simulink model "DV3A_String1_Diode"  (R2023b)
settings: Solver=VariableStepAuto  StartTime=0.0  StopTime=1  FixedStep=Ts_Power  MinStep=0.0025  RelTol=1e-4
PreLoadFcn:
  | Ts_Power=5e-4;
  | Slope_Vdc=1;
InitFcn:
  | Ts_Power=50e-6;
  | Tc=1e-5;%break algebraic loop time constant
StopFcn:
  | if exist('I','var') && exist('V','var')
  |    figure(1)
  |    clf
  |    n=find(I>=0);
  |    n=n(end);
  |    Vglobal=V(1:n);
  |    Iglobal=I(1:n);
  | 
  | 
  |    Pglobal=Vglobal.*Iglobal;
  |    n=find(Pglobal==max(Pglobal));
  |    Pmax=Pglobal(n);
  |    Vmp=Vglobal(n);
  |    Imp=Iglobal(n);
  | 
  | 
  |    subplot(211)
  |    plot(Vglobal, Iglobal,Vmp,Imp,'or')
  |    ylabel('Current (A)')
  |    title(sprintf('Global I-V & P-V characteristics\n %s' ,ModuleName))
  | 
  | 
  |    subplot(212)
  |    plot(Vglobal, Pglobal,Vmp,Pmax,'or')
  |    ylabel('Power (W)')
  |    xlabel('Voltage (V)')
  | end
model workspace (MAT data in the model file):
  slope_Vdc = 3.0848387096
undefined symbols (not defined in the file): Slope_Vdc_string1
libraries: spsPVArrayLib x142, spsVariableResistorLib x142, spsDiodeLib x29, spsCurrentMeasurementLib x1, spsVoltageMeasurementLib x1, spsControlledVoltageSourceLib x1, simulink x1, spspowerguiLib x1
(part 1 of 8)
settings Model: Creator=MathWorks  LastModifiedBy=IT
settings SolverCC: AlgebraicLoopSolver=LineSearch
settings DataIOCC: ExternalInput=[]  LimitDataPoints=on  LoadExternalInput=on  SaveFormat=Array  SaveOutput=off  SignalLogging=off  DSMLogging=off  SaveTime=off  ReturnWorkspaceOutputs=off
settings OptimizationCC: ExpressionDepthLimit=2147483647  LifeSpan=inf
settings DebuggingCC: UnderspecifiedInitializationDetection=Classic  MergeDetectMultiDrivingBlocksExec=none  SolverPrmCheckMsg=warning  FcnCallInpInsideContextMsg=warning  UnconnectedInputMsg=warning  UnconnectedOutputMsg=warning  UnconnectedLineMsg=warning  AllowSymbolicDim=off  StateNameClashWarn=warning  SFUnexpectedBacktrackingDiag=warning  SFNoUnconditionalDefaultTransitionDiag=warning  SFExecutionAtInitializationDiag=none  ArithmeticOperatorsInVariantConditions=warning
settings HardwareCC: ProdBitPerPointer=32  ProdBitPerSizeT=32  ProdBitPerPtrDiffT=32  ProdLargestAtomicFloat=None  ProdIntDivRoundTo=Undefined  ProdEndianess=Unspecified  ProdWordSize=32  ProdHWDeviceType=32-bit Generic
settings ModelReferenceCC: EnableRefExpFcnMdlSchedulingChecks=on  PropagateSignalLabelsOutOfModel=off
settings SFSimCC: SimUseLocalCustomCode=off  CustomCodeUndefinedFunction=UseInterfaceOnly
settings RTWCC: RTWUseLocalCustomCode=off  DLArmComputeVersion=19.05
settings CodeAppCC: StateflowObjectComments=on
settings GRTTargetCC: TargetLangStandard=C89/C90 (ANSI)  CombineOutputUpdateFcns=off  GRTInterface=on
settings ConfigComp: CovMetricSettings=dw  CovSaveCumulativeToWorkspaceVar=on  CovSaveSingleToWorkspaceVar=on  CovExternalEMLEnable=off  CovSFcnEnable=off
settings SimscapeCC: SimscapeNormalizeSystem=off

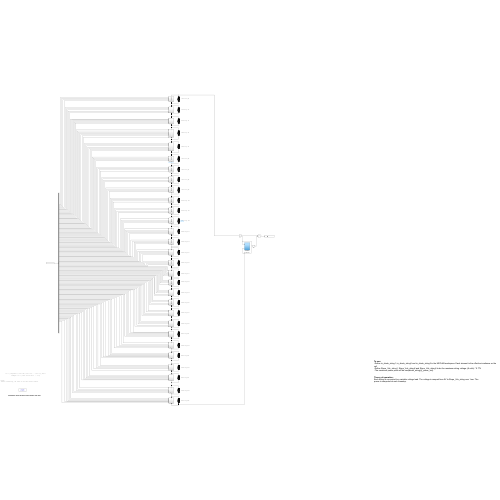
[thumbnail: Simulink's stored preview of the top-level diagram]
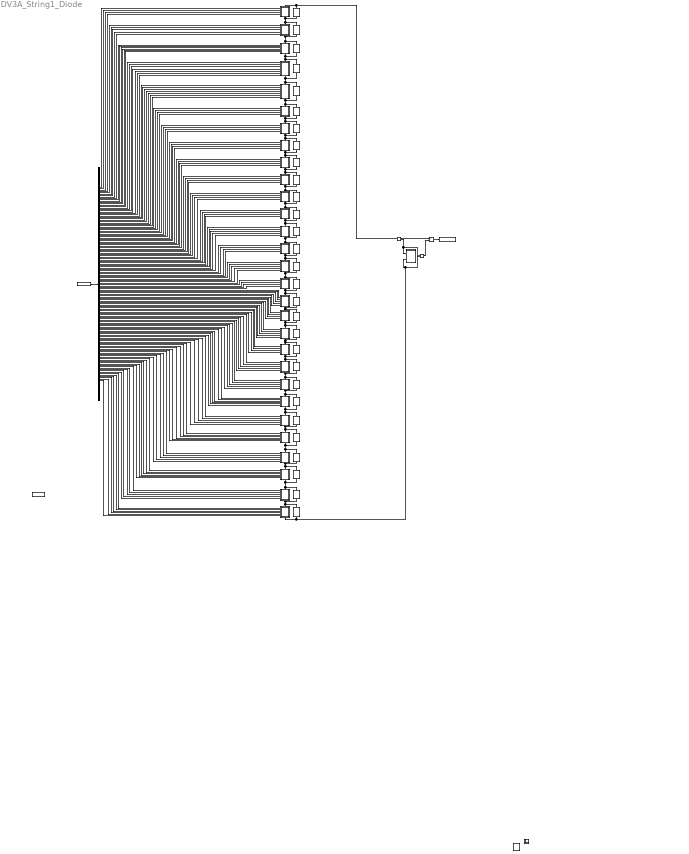
== system DV3A_String1_Diode ==
  note: irr = [(required 0) (cell 142) (cell 141) ... (cell 1)], W/m^2
  note: Notes:
      | -Within a substring, the order of the cells doesn't matter
  note: Final DV3A - String #1 with bypass diodes (142 cells)
  note: Example: irr = [0 800 700 242 573.3 ... 473]
  note: To use:
      | -Define irr_diode_string1, irr_diode_string2 and irr_diode_string3 in the MATLAB workspace. Each element is the effective irradiance on the cell
      | -Define Slope_Vdc_string1, Slope_Vdc_string2 and Slope_Vdc_string3 to be the maximum string voltage: (# cells) * 0.77V
      | -The maximum power point will be max(diode_string[n]_power_out )
  note: Theory of operation:
      | Each string is connected to a variable voltage load. The voltage is ramped from 0V to Slope_Vdc_string over 1sec. The power is computed at each timestep.
  note: Substring #1
  note: Substring #2
  note: Substring #3
  note: Substring #4
  note: Substring #5
  note: Substring #6
  note: Substring #7
  note: Substring #9
  note: Substring #8
  note: Substring #11
  note: Substring #10
  note: Substring #12
  note: Substring #13
  note: Substring #15
  note: Substring #14
  note: Substring #17
  note: Substring #16
  note: Substring #18
  note: Substring #19
  note: Substring #20
  note: Substring #21
  note: Substring #22
  note: Substring #23
  note: Substring #25
  note: Substring #24
  note: Substring #27
  note: Substring #26
  note: Substring #29
  note: Substring #28
  Bypass Diode {12..20,34..53} (29 alike) : spsDiodeLib/Diode  Ron=0.00333333  Lon=0  Vf=0.01993333134  IC=0  UseSnubber=off  Rs=1000000000  Cs=250e-15  Measurements=off
  Demux2 : Demux  Outputs=142
  From Workspace2 : FromWorkspace  VariableName=irr_diode_string_String1
  I1 : spsCurrentMeasurementLib/Current Measurement  PhasorSimulation=off  OutputType=Complex  PSBequivalent=0
  Product2 : Product
  Subsystem12 : Subsystem
      settings: PortSchema="{\"entries\":[{\"content\":{\"sides\":[{\"content\":{\"connectorIds\":[\"In1\",\"In2\",\"In3\",\"In4\"]},\"type\":\"ConnectorPlacement.EquallySpacedRectSide\",\"uuid\":\"ec6071b1-e44d-45a4-9204-34cda7b2c9be\"},{\"content\":{\"connectorIds\":[],\"side\":\"RIGHT\"},\"type\":\"ConnectorPlacement.EquallySpacedRectSide\",\"uuid\":\"8ac2ba72-278d-4942-985d-63a53d830fa7\"},{\"content\":{\"connectorIds\":[\"LConn1\"],\"side\":\"TOP\"},\"type\":\"ConnectorPlacement.EquallySpacedRectSide\",\"uuid\":\"91abef48-6106-4bba-9094-b5b4c6d4927b\"},{\"content\":{\"connectorIds\":[\"RConn1\"],\"side\":\"BOTTOM\"},\"type\":\"ConnectorPlacement.EquallySpacedRectSide\",\"uuid\":\"2339e630-2664-445f-8cd2-24ead5b760e5\"}]},\"type\":\"ConnectorPlacement.EquallySpacedConnector\",\"uuid\":\"6b30c10d-3aac-43c1-96cb-d205f04f2f88\"}],\"packageUris\":[\"http://schema.mathworks.com/mf0/Connector/R2020b\"],\"version\":\"1.0\"}"
  Subsystem13 : Subsystem
      settings: PortSchema="{\"entries\":[{\"content\":{\"sides\":[{\"content\":{\"connectorIds\":[\"In1\",\"In2\",\"In3\",\"In4\",\"In5\"]},\"type\":\"ConnectorPlacement.EquallySpacedRectSide\",\"uuid\":\"ec6071b1-e44d-45a4-9204-34cda7b2c9be\"},{\"content\":{\"side\":\"RIGHT\"},\"type\":\"ConnectorPlacement.EquallySpacedRectSide\",\"uuid\":\"8ac2ba72-278d-4942-985d-63a53d830fa7\"},{\"content\":{\"connectorIds\":[\"LConn1\"],\"side\":\"TOP\"},\"type\":\"ConnectorPlacement.EquallySpacedRectSide\",\"uuid\":\"91abef48-6106-4bba-9094-b5b4c6d4927b\"},{\"content\":{\"connectorIds\":[\"RConn1\"],\"side\":\"BOTTOM\"},\"type\":\"ConnectorPlacement.EquallySpacedRectSide\",\"uuid\":\"2339e630-2664-445f-8cd2-24ead5b760e5\"}]},\"type\":\"ConnectorPlacement.EquallySpacedConnector\",\"uuid\":\"6b30c10d-3aac-43c1-96cb-d205f04f2f88\"}],\"packageUris\":[\"http://schema.mathworks.com/mf0/Connector/R2020b\"],\"version\":\"1.0\"}"
  Subsystem14 : Subsystem
      settings: PortSchema="{\"entries\":[{\"content\":{\"sides\":[{\"content\":{\"connectorIds\":[\"In1\",\"In2\",\"In3\",\"In4\",\"In5\",\"In6\"]},\"type\":\"ConnectorPlacement.EquallySpacedRectSide\",\"uuid\":\"ec6071b1-e44d-45a4-9204-34cda7b2c9be\"},{\"content\":{\"side\":\"RIGHT\"},\"type\":\"ConnectorPlacement.EquallySpacedRectSide\",\"uuid\":\"8ac2ba72-278d-4942-985d-63a53d830fa7\"},{\"content\":{\"connectorIds\":[\"LConn1\"],\"side\":\"TOP\"},\"type\":\"ConnectorPlacement.EquallySpacedRectSide\",\"uuid\":\"91abef48-6106-4bba-9094-b5b4c6d4927b\"},{\"content\":{\"connectorIds\":[\"RConn1\"],\"side\":\"BOTTOM\"},\"type\":\"ConnectorPlacement.EquallySpacedRectSide\",\"uuid\":\"2339e630-2664-445f-8cd2-24ead5b760e5\"}]},\"type\":\"ConnectorPlacement.EquallySpacedConnector\",\"uuid\":\"6b30c10d-3aac-43c1-96cb-d205f04f2f88\"}],\"packageUris\":[\"http://schema.mathworks.com/mf0/Connector/R2020b\"],\"version\":\"1.0\"}"
  Subsystem15 : Subsystem
      settings: PortSchema="{\"entries\":[{\"content\":{\"sides\":[{\"content\":{\"connectorIds\":[\"In1\",\"In2\",\"In3\",\"In4\",\"In5\",\"In6\",\"In7\"]},\"type\":\"ConnectorPlacement.EquallySpacedRectSide\",\"uuid\":\"ec6071b1-e44d-45a4-9204-34cda7b2c9be\"},{\"content\":{\"connectorIds\":[],\"side\":\"RIGHT\"},\"type\":\"ConnectorPlacement.EquallySpacedRectSide\",\"uuid\":\"8ac2ba72-278d-4942-985d-63a53d830fa7\"},{\"content\":{\"connectorIds\":[\"LConn1\"],\"side\":\"TOP\"},\"type\":\"ConnectorPlacement.EquallySpacedRectSide\",\"uuid\":\"91abef48-6106-4bba-9094-b5b4c6d4927b\"},{\"content\":{\"connectorIds\":[\"RConn1\"],\"side\":\"BOTTOM\"},\"type\":\"ConnectorPlacement.EquallySpacedRectSide\",\"uuid\":\"2339e630-2664-445f-8cd2-24ead5b760e5\"}]},\"type\":\"ConnectorPlacement.EquallySpacedConnector\",\"uuid\":\"6b30c10d-3aac-43c1-96cb-d205f04f2f88\"}],\"packageUris\":[\"http://schema.mathworks.com/mf0/Connector/R2020b\"],\"version\":\"1.0\"}"
  Subsystem16 : Subsystem
      settings: PortSchema="{\"entries\":[{\"content\":{\"sides\":[{\"content\":{\"connectorIds\":[\"In1\",\"In2\",\"In3\",\"In4\",\"In5\",\"In6\",\"In7\"]},\"type\":\"ConnectorPlacement.EquallySpacedRectSide\",\"uuid\":\"ec6071b1-e44d-45a4-9204-34cda7b2c9be\"},{\"content\":{\"connectorIds\":[],\"side\":\"RIGHT\"},\"type\":\"ConnectorPlacement.EquallySpacedRectSide\",\"uuid\":\"8ac2ba72-278d-4942-985d-63a53d830fa7\"},{\"content\":{\"connectorIds\":[\"LConn1\"],\"side\":\"TOP\"},\"type\":\"ConnectorPlacement.EquallySpacedRectSide\",\"uuid\":\"91abef48-6106-4bba-9094-b5b4c6d4927b\"},{\"content\":{\"connectorIds\":[\"RConn1\"],\"side\":\"BOTTOM\"},\"type\":\"ConnectorPlacement.EquallySpacedRectSide\",\"uuid\":\"2339e630-2664-445f-8cd2-24ead5b760e5\"}]},\"type\":\"ConnectorPlacement.EquallySpacedConnector\",\"uuid\":\"6b30c10d-3aac-43c1-96cb-d205f04f2f88\"}],\"packageUris\":[\"http://schema.mathworks.com/mf0/Connector/R2020b\"],\"version\":\"1.0\"}"
  Subsystem17 : Subsystem
      settings: PortSchema="{\"entries\":[{\"content\":{\"sides\":[{\"content\":{\"connectorIds\":[\"In1\",\"In2\",\"In3\",\"In4\"]},\"type\":\"ConnectorPlacement.EquallySpacedRectSide\",\"uuid\":\"ec6071b1-e44d-45a4-9204-34cda7b2c9be\"},{\"content\":{\"connectorIds\":[],\"side\":\"RIGHT\"},\"type\":\"ConnectorPlacement.EquallySpacedRectSide\",\"uuid\":\"8ac2ba72-278d-4942-985d-63a53d830fa7\"},{\"content\":{\"connectorIds\":[\"LConn1\"],\"side\":\"TOP\"},\"type\":\"ConnectorPlacement.EquallySpacedRectSide\",\"uuid\":\"91abef48-6106-4bba-9094-b5b4c6d4927b\"},{\"content\":{\"connectorIds\":[\"RConn1\"],\"side\":\"BOTTOM\"},\"type\":\"ConnectorPlacement.EquallySpacedRectSide\",\"uuid\":\"2339e630-2664-445f-8cd2-24ead5b760e5\"}]},\"type\":\"ConnectorPlacement.EquallySpacedConnector\",\"uuid\":\"6b30c10d-3aac-43c1-96cb-d205f04f2f88\"}],\"packageUris\":[\"http://schema.mathworks.com/mf0/Connector/R2020b\"],\"version\":\"1.0\"}"
  Subsystem18 : Subsystem
      settings: PortSchema="{\"entries\":[{\"content\":{\"sides\":[{\"content\":{\"connectorIds\":[\"In1\",\"In2\",\"In3\",\"In4\"]},\"type\":\"ConnectorPlacement.EquallySpacedRectSide\",\"uuid\":\"ec6071b1-e44d-45a4-9204-34cda7b2c9be\"},{\"content\":{\"connectorIds\":[],\"side\":\"RIGHT\"},\"type\":\"ConnectorPlacement.EquallySpacedRectSide\",\"uuid\":\"8ac2ba72-278d-4942-985d-63a53d830fa7\"},{\"content\":{\"connectorIds\":[\"LConn1\"],\"side\":\"TOP\"},\"type\":\"ConnectorPlacement.EquallySpacedRectSide\",\"uuid\":\"91abef48-6106-4bba-9094-b5b4c6d4927b\"},{\"content\":{\"connectorIds\":[\"RConn1\"],\"side\":\"BOTTOM\"},\"type\":\"ConnectorPlacement.EquallySpacedRectSide\",\"uuid\":\"2339e630-2664-445f-8cd2-24ead5b760e5\"}]},\"type\":\"ConnectorPlacement.EquallySpacedConnector\",\"uuid\":\"6b30c10d-3aac-43c1-96cb-d205f04f2f88\"}],\"packageUris\":[\"http://schema.mathworks.com/mf0/Connector/R2020b\"],\"version\":\"1.0\"}"
  Subsystem19 : Subsystem
      settings: PortSchema="{\"entries\":[{\"content\":{\"sides\":[{\"content\":{\"connectorIds\":[\"In1\",\"In2\",\"In3\",\"In4\"]},\"type\":\"ConnectorPlacement.EquallySpacedRectSide\",\"uuid\":\"ec6071b1-e44d-45a4-9204-34cda7b2c9be\"},{\"content\":{\"connectorIds\":[],\"side\":\"RIGHT\"},\"type\":\"ConnectorPlacement.EquallySpacedRectSide\",\"uuid\":\"8ac2ba72-278d-4942-985d-63a53d830fa7\"},{\"content\":{\"connectorIds\":[\"LConn1\"],\"side\":\"TOP\"},\"type\":\"ConnectorPlacement.EquallySpacedRectSide\",\"uuid\":\"91abef48-6106-4bba-9094-b5b4c6d4927b\"},{\"content\":{\"connectorIds\":[\"RConn1\"],\"side\":\"BOTTOM\"},\"type\":\"ConnectorPlacement.EquallySpacedRectSide\",\"uuid\":\"2339e630-2664-445f-8cd2-24ead5b760e5\"}]},\"type\":\"ConnectorPlacement.EquallySpacedConnector\",\"uuid\":\"6b30c10d-3aac-43c1-96cb-d205f04f2f88\"}],\"packageUris\":[\"http://schema.mathworks.com/mf0/Connector/R2020b\"],\"version\":\"1.0\"}"
  Subsystem20 : Subsystem
      settings: PortSchema="{\"entries\":[{\"content\":{\"sides\":[{\"content\":{\"connectorIds\":[\"In1\",\"In2\",\"In3\",\"In4\"]},\"type\":\"ConnectorPlacement.EquallySpacedRectSide\",\"uuid\":\"ec6071b1-e44d-45a4-9204-34cda7b2c9be\"},{\"content\":{\"connectorIds\":[],\"side\":\"RIGHT\"},\"type\":\"ConnectorPlacement.EquallySpacedRectSide\",\"uuid\":\"8ac2ba72-278d-4942-985d-63a53d830fa7\"},{\"content\":{\"connectorIds\":[\"LConn1\"],\"side\":\"TOP\"},\"type\":\"ConnectorPlacement.EquallySpacedRectSide\",\"uuid\":\"91abef48-6106-4bba-9094-b5b4c6d4927b\"},{\"content\":{\"connectorIds\":[\"RConn1\"],\"side\":\"BOTTOM\"},\"type\":\"ConnectorPlacement.EquallySpacedRectSide\",\"uuid\":\"2339e630-2664-445f-8cd2-24ead5b760e5\"}]},\"type\":\"ConnectorPlacement.EquallySpacedConnector\",\"uuid\":\"6b30c10d-3aac-43c1-96cb-d205f04f2f88\"}],\"packageUris\":[\"http://schema.mathworks.com/mf0/Connector/R2020b\"],\"version\":\"1.0\"}"
  Subsystem34 : Subsystem
      settings: PortSchema="{\"entries\":[{\"content\":{\"sides\":[{\"content\":{\"connectorIds\":[\"In1\",\"In2\",\"In3\",\"In4\"]},\"type\":\"ConnectorPlacement.EquallySpacedRectSide\",\"uuid\":\"ec6071b1-e44d-45a4-9204-34cda7b2c9be\"},{\"content\":{\"connectorIds\":[],\"side\":\"RIGHT\"},\"type\":\"ConnectorPlacement.EquallySpacedRectSide\",\"uuid\":\"8ac2ba72-278d-4942-985d-63a53d830fa7\"},{\"content\":{\"connectorIds\":[\"LConn1\"],\"side\":\"TOP\"},\"type\":\"ConnectorPlacement.EquallySpacedRectSide\",\"uuid\":\"91abef48-6106-4bba-9094-b5b4c6d4927b\"},{\"content\":{\"connectorIds\":[\"RConn1\"],\"side\":\"BOTTOM\"},\"type\":\"ConnectorPlacement.EquallySpacedRectSide\",\"uuid\":\"2339e630-2664-445f-8cd2-24ead5b760e5\"}]},\"type\":\"ConnectorPlacement.EquallySpacedConnector\",\"uuid\":\"6b30c10d-3aac-43c1-96cb-d205f04f2f88\"}],\"packageUris\":[\"http://schema.mathworks.com/mf0/Connector/R2020b\"],\"version\":\"1.0\"}"
  Subsystem35 : Subsystem
      settings: PortSchema="{\"entries\":[{\"content\":{\"sides\":[{\"content\":{\"connectorIds\":[\"In1\",\"In2\",\"In3\",\"In4\"]},\"type\":\"ConnectorPlacement.EquallySpacedRectSide\",\"uuid\":\"ec6071b1-e44d-45a4-9204-34cda7b2c9be\"},{\"content\":{\"connectorIds\":[],\"side\":\"RIGHT\"},\"type\":\"ConnectorPlacement.EquallySpacedRectSide\",\"uuid\":\"8ac2ba72-278d-4942-985d-63a53d830fa7\"},{\"content\":{\"connectorIds\":[\"LConn1\"],\"side\":\"TOP\"},\"type\":\"ConnectorPlacement.EquallySpacedRectSide\",\"uuid\":\"91abef48-6106-4bba-9094-b5b4c6d4927b\"},{\"content\":{\"connectorIds\":[\"RConn1\"],\"side\":\"BOTTOM\"},\"type\":\"ConnectorPlacement.EquallySpacedRectSide\",\"uuid\":\"2339e630-2664-445f-8cd2-24ead5b760e5\"}]},\"type\":\"ConnectorPlacement.EquallySpacedConnector\",\"uuid\":\"6b30c10d-3aac-43c1-96cb-d205f04f2f88\"}],\"packageUris\":[\"http://schema.mathworks.com/mf0/Connector/R2020b\"],\"version\":\"1.0\"}"
  Subsystem36 : Subsystem
      settings: PortSchema="{\"entries\":[{\"content\":{\"sides\":[{\"content\":{\"connectorIds\":[\"In1\",\"In2\",\"In3\",\"In4\"]},\"type\":\"ConnectorPlacement.EquallySpacedRectSide\",\"uuid\":\"ec6071b1-e44d-45a4-9204-34cda7b2c9be\"},{\"content\":{\"connectorIds\":[],\"side\":\"RIGHT\"},\"type\":\"ConnectorPlacement.EquallySpacedRectSide\",\"uuid\":\"8ac2ba72-278d-4942-985d-63a53d830fa7\"},{\"content\":{\"connectorIds\":[\"LConn1\"],\"side\":\"TOP\"},\"type\":\"ConnectorPlacement.EquallySpacedRectSide\",\"uuid\":\"91abef48-6106-4bba-9094-b5b4c6d4927b\"},{\"content\":{\"connectorIds\":[\"RConn1\"],\"side\":\"BOTTOM\"},\"type\":\"ConnectorPlacement.EquallySpacedRectSide\",\"uuid\":\"2339e630-2664-445f-8cd2-24ead5b760e5\"}]},\"type\":\"ConnectorPlacement.EquallySpacedConnector\",\"uuid\":\"6b30c10d-3aac-43c1-96cb-d205f04f2f88\"}],\"packageUris\":[\"http://schema.mathworks.com/mf0/Connector/R2020b\"],\"version\":\"1.0\"}"
  Subsystem37 : Subsystem
      settings: PortSchema="{\"entries\":[{\"content\":{\"sides\":[{\"content\":{\"connectorIds\":[\"In1\",\"In2\",\"In3\",\"In4\",\"In5\"]},\"type\":\"ConnectorPlacement.EquallySpacedRectSide\",\"uuid\":\"ec6071b1-e44d-45a4-9204-34cda7b2c9be\"},{\"content\":{\"side\":\"RIGHT\"},\"type\":\"ConnectorPlacement.EquallySpacedRectSide\",\"uuid\":\"8ac2ba72-278d-4942-985d-63a53d830fa7\"},{\"content\":{\"connectorIds\":[\"LConn1\"],\"side\":\"TOP\"},\"type\":\"ConnectorPlacement.EquallySpacedRectSide\",\"uuid\":\"91abef48-6106-4bba-9094-b5b4c6d4927b\"},{\"content\":{\"connectorIds\":[\"RConn1\"],\"side\":\"BOTTOM\"},\"type\":\"ConnectorPlacement.EquallySpacedRectSide\",\"uuid\":\"2339e630-2664-445f-8cd2-24ead5b760e5\"}]},\"type\":\"ConnectorPlacement.EquallySpacedConnector\",\"uuid\":\"6b30c10d-3aac-43c1-96cb-d205f04f2f88\"}],\"packageUris\":[\"http://schema.mathworks.com/mf0/Connector/R2020b\"],\"version\":\"1.0\"}"
  Subsystem38 : Subsystem
      settings: PortSchema="{\"entries\":[{\"content\":{\"sides\":[{\"content\":{\"connectorIds\":[\"In1\",\"In2\",\"In3\",\"In4\"]},\"type\":\"ConnectorPlacement.EquallySpacedRectSide\",\"uuid\":\"ec6071b1-e44d-45a4-9204-34cda7b2c9be\"},{\"content\":{\"connectorIds\":[],\"side\":\"RIGHT\"},\"type\":\"ConnectorPlacement.EquallySpacedRectSide\",\"uuid\":\"8ac2ba72-278d-4942-985d-63a53d830fa7\"},{\"content\":{\"connectorIds\":[\"LConn1\"],\"side\":\"TOP\"},\"type\":\"ConnectorPlacement.EquallySpacedRectSide\",\"uuid\":\"91abef48-6106-4bba-9094-b5b4c6d4927b\"},{\"content\":{\"connectorIds\":[\"RConn1\"],\"side\":\"BOTTOM\"},\"type\":\"ConnectorPlacement.EquallySpacedRectSide\",\"uuid\":\"2339e630-2664-445f-8cd2-24ead5b760e5\"}]},\"type\":\"ConnectorPlacement.EquallySpacedConnector\",\"uuid\":\"6b30c10d-3aac-43c1-96cb-d205f04f2f88\"}],\"packageUris\":[\"http://schema.mathworks.com/mf0/Connector/R2020b\"],\"version\":\"1.0\"}"
  Subsystem39 : Subsystem
      settings: PortSchema="{\"entries\":[{\"content\":{\"sides\":[{\"content\":{\"connectorIds\":[\"In1\",\"In2\",\"In3\",\"In4\",\"In5\"]},\"type\":\"ConnectorPlacement.EquallySpacedRectSide\",\"uuid\":\"ec6071b1-e44d-45a4-9204-34cda7b2c9be\"},{\"content\":{\"side\":\"RIGHT\"},\"type\":\"ConnectorPlacement.EquallySpacedRectSide\",\"uuid\":\"8ac2ba72-278d-4942-985d-63a53d830fa7\"},{\"content\":{\"connectorIds\":[\"LConn1\"],\"side\":\"TOP\"},\"type\":\"ConnectorPlacement.EquallySpacedRectSide\",\"uuid\":\"91abef48-6106-4bba-9094-b5b4c6d4927b\"},{\"content\":{\"connectorIds\":[\"RConn1\"],\"side\":\"BOTTOM\"},\"type\":\"ConnectorPlacement.EquallySpacedRectSide\",\"uuid\":\"2339e630-2664-445f-8cd2-24ead5b760e5\"}]},\"type\":\"ConnectorPlacement.EquallySpacedConnector\",\"uuid\":\"6b30c10d-3aac-43c1-96cb-d205f04f2f88\"}],\"packageUris\":[\"http://schema.mathworks.com/mf0/Connector/R2020b\"],\"version\":\"1.0\"}"
  Subsystem40 : Subsystem
      settings: PortSchema="{\"entries\":[{\"content\":{\"sides\":[{\"content\":{\"connectorIds\":[\"In1\",\"In2\",\"In3\",\"In4\"]},\"type\":\"ConnectorPlacement.EquallySpacedRectSide\",\"uuid\":\"ec6071b1-e44d-45a4-9204-34cda7b2c9be\"},{\"content\":{\"connectorIds\":[],\"side\":\"RIGHT\"},\"type\":\"ConnectorPlacement.EquallySpacedRectSide\",\"uuid\":\"8ac2ba72-278d-4942-985d-63a53d830fa7\"},{\"content\":{\"connectorIds\":[\"LConn1\"],\"side\":\"TOP\"},\"type\":\"ConnectorPlacement.EquallySpacedRectSide\",\"uuid\":\"91abef48-6106-4bba-9094-b5b4c6d4927b\"},{\"content\":{\"connectorIds\":[\"RConn1\"],\"side\":\"BOTTOM\"},\"type\":\"ConnectorPlacement.EquallySpacedRectSide\",\"uuid\":\"2339e630-2664-445f-8cd2-24ead5b760e5\"}]},\"type\":\"ConnectorPlacement.EquallySpacedConnector\",\"uuid\":\"6b30c10d-3aac-43c1-96cb-d205f04f2f88\"}],\"packageUris\":[\"http://schema.mathworks.com/mf0/Connector/R2020b\"],\"version\":\"1.0\"}"
  Subsystem41 : Subsystem
      settings: PortSchema="{\"entries\":[{\"content\":{\"sides\":[{\"content\":{\"connectorIds\":[\"In1\",\"In2\",\"In3\",\"In4\",\"In5\"]},\"type\":\"ConnectorPlacement.EquallySpacedRectSide\",\"uuid\":\"ec6071b1-e44d-45a4-9204-34cda7b2c9be\"},{\"content\":{\"side\":\"RIGHT\"},\"type\":\"ConnectorPlacement.EquallySpacedRectSide\",\"uuid\":\"8ac2ba72-278d-4942-985d-63a53d830fa7\"},{\"content\":{\"connectorIds\":[\"LConn1\"],\"side\":\"TOP\"},\"type\":\"ConnectorPlacement.EquallySpacedRectSide\",\"uuid\":\"91abef48-6106-4bba-9094-b5b4c6d4927b\"},{\"content\":{\"connectorIds\":[\"RConn1\"],\"side\":\"BOTTOM\"},\"type\":\"ConnectorPlacement.EquallySpacedRectSide\",\"uuid\":\"2339e630-2664-445f-8cd2-24ead5b760e5\"}]},\"type\":\"ConnectorPlacement.EquallySpacedConnector\",\"uuid\":\"6b30c10d-3aac-43c1-96cb-d205f04f2f88\"}],\"packageUris\":[\"http://schema.mathworks.com/mf0/Connector/R2020b\"],\"version\":\"1.0\"}"
  Subsystem42 : Subsystem
      settings: PortSchema="{\"entries\":[{\"content\":{\"sides\":[{\"content\":{\"connectorIds\":[\"In1\",\"In2\",\"In3\",\"In4\"]},\"type\":\"ConnectorPlacement.EquallySpacedRectSide\",\"uuid\":\"ec6071b1-e44d-45a4-9204-34cda7b2c9be\"},{\"content\":{\"connectorIds\":[],\"side\":\"RIGHT\"},\"type\":\"ConnectorPlacement.EquallySpacedRectSide\",\"uuid\":\"8ac2ba72-278d-4942-985d-63a53d830fa7\"},{\"content\":{\"connectorIds\":[\"LConn1\"],\"side\":\"TOP\"},\"type\":\"ConnectorPlacement.EquallySpacedRectSide\",\"uuid\":\"91abef48-6106-4bba-9094-b5b4c6d4927b\"},{\"content\":{\"connectorIds\":[\"RConn1\"],\"side\":\"BOTTOM\"},\"type\":\"ConnectorPlacement.EquallySpacedRectSide\",\"uuid\":\"2339e630-2664-445f-8cd2-24ead5b760e5\"}]},\"type\":\"ConnectorPlacement.EquallySpacedConnector\",\"uuid\":\"6b30c10d-3aac-43c1-96cb-d205f04f2f88\"}],\"packageUris\":[\"http://schema.mathworks.com/mf0/Connector/R2020b\"],\"version\":\"1.0\"}"
  Subsystem43 : Subsystem
      settings: PortSchema="{\"entries\":[{\"content\":{\"sides\":[{\"content\":{\"connectorIds\":[\"In1\",\"In2\",\"In3\",\"In4\",\"In5\"]},\"type\":\"ConnectorPlacement.EquallySpacedRectSide\",\"uuid\":\"ec6071b1-e44d-45a4-9204-34cda7b2c9be\"},{\"content\":{\"side\":\"RIGHT\"},\"type\":\"ConnectorPlacement.EquallySpacedRectSide\",\"uuid\":\"8ac2ba72-278d-4942-985d-63a53d830fa7\"},{\"content\":{\"connectorIds\":[\"LConn1\"],\"side\":\"TOP\"},\"type\":\"ConnectorPlacement.EquallySpacedRectSide\",\"uuid\":\"91abef48-6106-4bba-9094-b5b4c6d4927b\"},{\"content\":{\"connectorIds\":[\"RConn1\"],\"side\":\"BOTTOM\"},\"type\":\"ConnectorPlacement.EquallySpacedRectSide\",\"uuid\":\"2339e630-2664-445f-8cd2-24ead5b760e5\"}]},\"type\":\"ConnectorPlacement.EquallySpacedConnector\",\"uuid\":\"6b30c10d-3aac-43c1-96cb-d205f04f2f88\"}],\"packageUris\":[\"http://schema.mathworks.com/mf0/Connector/R2020b\"],\"version\":\"1.0\"}"
  Subsystem44 : Subsystem
      settings: PortSchema="{\"entries\":[{\"content\":{\"sides\":[{\"content\":{\"connectorIds\":[\"In1\",\"In2\",\"In3\",\"In4\"]},\"type\":\"ConnectorPlacement.EquallySpacedRectSide\",\"uuid\":\"ec6071b1-e44d-45a4-9204-34cda7b2c9be\"},{\"content\":{\"connectorIds\":[],\"side\":\"RIGHT\"},\"type\":\"ConnectorPlacement.EquallySpacedRectSide\",\"uuid\":\"8ac2ba72-278d-4942-985d-63a53d830fa7\"},{\"content\":{\"connectorIds\":[\"LConn1\"],\"side\":\"TOP\"},\"type\":\"ConnectorPlacement.EquallySpacedRectSide\",\"uuid\":\"91abef48-6106-4bba-9094-b5b4c6d4927b\"},{\"content\":{\"connectorIds\":[\"RConn1\"],\"side\":\"BOTTOM\"},\"type\":\"ConnectorPlacement.EquallySpacedRectSide\",\"uuid\":\"2339e630-2664-445f-8cd2-24ead5b760e5\"}]},\"type\":\"ConnectorPlacement.EquallySpacedConnector\",\"uuid\":\"6b30c10d-3aac-43c1-96cb-d205f04f2f88\"}],\"packageUris\":[\"http://schema.mathworks.com/mf0/Connector/R2020b\"],\"version\":\"1.0\"}"
  Subsystem45 : Subsystem
      settings: PortSchema="{\"entries\":[{\"content\":{\"sides\":[{\"content\":{\"connectorIds\":[\"In1\",\"In2\",\"In3\",\"In4\",\"In5\"]},\"type\":\"ConnectorPlacement.EquallySpacedRectSide\",\"uuid\":\"ec6071b1-e44d-45a4-9204-34cda7b2c9be\"},{\"content\":{\"side\":\"RIGHT\"},\"type\":\"ConnectorPlacement.EquallySpacedRectSide\",\"uuid\":\"8ac2ba72-278d-4942-985d-63a53d830fa7\"},{\"content\":{\"connectorIds\":[\"LConn1\"],\"side\":\"TOP\"},\"type\":\"ConnectorPlacement.EquallySpacedRectSide\",\"uuid\":\"91abef48-6106-4bba-9094-b5b4c6d4927b\"},{\"content\":{\"connectorIds\":[\"RConn1\"],\"side\":\"BOTTOM\"},\"type\":\"ConnectorPlacement.EquallySpacedRectSide\",\"uuid\":\"2339e630-2664-445f-8cd2-24ead5b760e5\"}]},\"type\":\"ConnectorPlacement.EquallySpacedConnector\",\"uuid\":\"6b30c10d-3aac-43c1-96cb-d205f04f2f88\"}],\"packageUris\":[\"http://schema.mathworks.com/mf0/Connector/R2020b\"],\"version\":\"1.0\"}"
  Subsystem46 : Subsystem
      settings: PortSchema="{\"entries\":[{\"content\":{\"sides\":[{\"content\":{\"connectorIds\":[\"In1\",\"In2\",\"In3\",\"In4\",\"In5\"]},\"type\":\"ConnectorPlacement.EquallySpacedRectSide\",\"uuid\":\"ec6071b1-e44d-45a4-9204-34cda7b2c9be\"},{\"content\":{\"side\":\"RIGHT\"},\"type\":\"ConnectorPlacement.EquallySpacedRectSide\",\"uuid\":\"8ac2ba72-278d-4942-985d-63a53d830fa7\"},{\"content\":{\"connectorIds\":[\"LConn1\"],\"side\":\"TOP\"},\"type\":\"ConnectorPlacement.EquallySpacedRectSide\",\"uuid\":\"91abef48-6106-4bba-9094-b5b4c6d4927b\"},{\"content\":{\"connectorIds\":[\"RConn1\"],\"side\":\"BOTTOM\"},\"type\":\"ConnectorPlacement.EquallySpacedRectSide\",\"uuid\":\"2339e630-2664-445f-8cd2-24ead5b760e5\"}]},\"type\":\"ConnectorPlacement.EquallySpacedConnector\",\"uuid\":\"6b30c10d-3aac-43c1-96cb-d205f04f2f88\"}],\"packageUris\":[\"http://schema.mathworks.com/mf0/Connector/R2020b\"],\"version\":\"1.0\"}"
  Subsystem47 : Subsystem
      settings: PortSchema="{\"entries\":[{\"content\":{\"sides\":[{\"content\":{\"connectorIds\":[\"In1\",\"In2\",\"In3\",\"In4\",\"In5\",\"In6\"]},\"type\":\"ConnectorPlacement.EquallySpacedRectSide\",\"uuid\":\"ec6071b1-e44d-45a4-9204-34cda7b2c9be\"},{\"content\":{\"side\":\"RIGHT\"},\"type\":\"ConnectorPlacement.EquallySpacedRectSide\",\"uuid\":\"8ac2ba72-278d-4942-985d-63a53d830fa7\"},{\"content\":{\"connectorIds\":[\"LConn1\"],\"side\":\"TOP\"},\"type\":\"ConnectorPlacement.EquallySpacedRectSide\",\"uuid\":\"91abef48-6106-4bba-9094-b5b4c6d4927b\"},{\"content\":{\"connectorIds\":[\"RConn1\"],\"side\":\"BOTTOM\"},\"type\":\"ConnectorPlacement.EquallySpacedRectSide\",\"uuid\":\"2339e630-2664-445f-8cd2-24ead5b760e5\"}]},\"type\":\"ConnectorPlacement.EquallySpacedConnector\",\"uuid\":\"6b30c10d-3aac-43c1-96cb-d205f04f2f88\"}],\"packageUris\":[\"http://schema.mathworks.com/mf0/Connector/R2020b\"],\"version\":\"1.0\"}"
  Subsystem48 : Subsystem
      settings: PortSchema="{\"entries\":[{\"content\":{\"sides\":[{\"content\":{\"connectorIds\":[\"In1\",\"In2\",\"In3\",\"In4\",\"In5\"]},\"type\":\"ConnectorPlacement.EquallySpacedRectSide\",\"uuid\":\"ec6071b1-e44d-45a4-9204-34cda7b2c9be\"},{\"content\":{\"side\":\"RIGHT\"},\"type\":\"ConnectorPlacement.EquallySpacedRectSide\",\"uuid\":\"8ac2ba72-278d-4942-985d-63a53d830fa7\"},{\"content\":{\"connectorIds\":[\"LConn1\"],\"side\":\"TOP\"},\"type\":\"ConnectorPlacement.EquallySpacedRectSide\",\"uuid\":\"91abef48-6106-4bba-9094-b5b4c6d4927b\"},{\"content\":{\"connectorIds\":[\"RConn1\"],\"side\":\"BOTTOM\"},\"type\":\"ConnectorPlacement.EquallySpacedRectSide\",\"uuid\":\"2339e630-2664-445f-8cd2-24ead5b760e5\"}]},\"type\":\"ConnectorPlacement.EquallySpacedConnector\",\"uuid\":\"6b30c10d-3aac-43c1-96cb-d205f04f2f88\"}],\"packageUris\":[\"http://schema.mathworks.com/mf0/Connector/R2020b\"],\"version\":\"1.0\"}"
  Subsystem49 : Subsystem
      settings: PortSchema="{\"entries\":[{\"content\":{\"sides\":[{\"content\":{\"connectorIds\":[\"In1\",\"In2\",\"In3\",\"In4\",\"In5\",\"In6\"]},\"type\":\"ConnectorPlacement.EquallySpacedRectSide\",\"uuid\":\"ec6071b1-e44d-45a4-9204-34cda7b2c9be\"},{\"content\":{\"side\":\"RIGHT\"},\"type\":\"ConnectorPlacement.EquallySpacedRectSide\",\"uuid\":\"8ac2ba72-278d-4942-985d-63a53d830fa7\"},{\"content\":{\"connectorIds\":[\"LConn1\"],\"side\":\"TOP\"},\"type\":\"ConnectorPlacement.EquallySpacedRectSide\",\"uuid\":\"91abef48-6106-4bba-9094-b5b4c6d4927b\"},{\"content\":{\"connectorIds\":[\"RConn1\"],\"side\":\"BOTTOM\"},\"type\":\"ConnectorPlacement.EquallySpacedRectSide\",\"uuid\":\"2339e630-2664-445f-8cd2-24ead5b760e5\"}]},\"type\":\"ConnectorPlacement.EquallySpacedConnector\",\"uuid\":\"6b30c10d-3aac-43c1-96cb-d205f04f2f88\"}],\"packageUris\":[\"http://schema.mathworks.com/mf0/Connector/R2020b\"],\"version\":\"1.0\"}"
  Subsystem50 : Subsystem
      settings: PortSchema="{\"entries\":[{\"content\":{\"sides\":[{\"content\":{\"connectorIds\":[\"In1\",\"In2\",\"In3\",\"In4\",\"In5\"]},\"type\":\"ConnectorPlacement.EquallySpacedRectSide\",\"uuid\":\"ec6071b1-e44d-45a4-9204-34cda7b2c9be\"},{\"content\":{\"side\":\"RIGHT\"},\"type\":\"ConnectorPlacement.EquallySpacedRectSide\",\"uuid\":\"8ac2ba72-278d-4942-985d-63a53d830fa7\"},{\"content\":{\"connectorIds\":[\"LConn1\"],\"side\":\"TOP\"},\"type\":\"ConnectorPlacement.EquallySpacedRectSide\",\"uuid\":\"91abef48-6106-4bba-9094-b5b4c6d4927b\"},{\"content\":{\"connectorIds\":[\"RConn1\"],\"side\":\"BOTTOM\"},\"type\":\"ConnectorPlacement.EquallySpacedRectSide\",\"uuid\":\"2339e630-2664-445f-8cd2-24ead5b760e5\"}]},\"type\":\"ConnectorPlacement.EquallySpacedConnector\",\"uuid\":\"6b30c10d-3aac-43c1-96cb-d205f04f2f88\"}],\"packageUris\":[\"http://schema.mathworks.com/mf0/Connector/R2020b\"],\"version\":\"1.0\"}"
  Subsystem51 : Subsystem
      settings: PortSchema="{\"entries\":[{\"content\":{\"sides\":[{\"content\":{\"connectorIds\":[\"In1\",\"In2\",\"In3\",\"In4\",\"In5\",\"In6\"]},\"type\":\"ConnectorPlacement.EquallySpacedRectSide\",\"uuid\":\"ec6071b1-e44d-45a4-9204-34cda7b2c9be\"},{\"content\":{\"side\":\"RIGHT\"},\"type\":\"ConnectorPlacement.EquallySpacedRectSide\",\"uuid\":\"8ac2ba72-278d-4942-985d-63a53d830fa7\"},{\"content\":{\"connectorIds\":[\"LConn1\"],\"side\":\"TOP\"},\"type\":\"ConnectorPlacement.EquallySpacedRectSide\",\"uuid\":\"91abef48-6106-4bba-9094-b5b4c6d4927b\"},{\"content\":{\"connectorIds\":[\"RConn1\"],\"side\":\"BOTTOM\"},\"type\":\"ConnectorPlacement.EquallySpacedRectSide\",\"uuid\":\"2339e630-2664-445f-8cd2-24ead5b760e5\"}]},\"type\":\"ConnectorPlacement.EquallySpacedConnector\",\"uuid\":\"6b30c10d-3aac-43c1-96cb-d205f04f2f88\"}],\"packageUris\":[\"http://schema.mathworks.com/mf0/Connector/R2020b\"],\"version\":\"1.0\"}"
  Subsystem52 : Subsystem
      settings: PortSchema="{\"entries\":[{\"content\":{\"sides\":[{\"content\":{\"connectorIds\":[\"In1\",\"In2\",\"In3\",\"In4\",\"In5\"]},\"type\":\"ConnectorPlacement.EquallySpacedRectSide\",\"uuid\":\"ec6071b1-e44d-45a4-9204-34cda7b2c9be\"},{\"content\":{\"side\":\"RIGHT\"},\"type\":\"ConnectorPlacement.EquallySpacedRectSide\",\"uuid\":\"8ac2ba72-278d-4942-985d-63a53d830fa7\"},{\"content\":{\"connectorIds\":[\"LConn1\"],\"side\":\"TOP\"},\"type\":\"ConnectorPlacement.EquallySpacedRectSide\",\"uuid\":\"91abef48-6106-4bba-9094-b5b4c6d4927b\"},{\"content\":{\"connectorIds\":[\"RConn1\"],\"side\":\"BOTTOM\"},\"type\":\"ConnectorPlacement.EquallySpacedRectSide\",\"uuid\":\"2339e630-2664-445f-8cd2-24ead5b760e5\"}]},\"type\":\"ConnectorPlacement.EquallySpacedConnector\",\"uuid\":\"6b30c10d-3aac-43c1-96cb-d205f04f2f88\"}],\"packageUris\":[\"http://schema.mathworks.com/mf0/Connector/R2020b\"],\"version\":\"1.0\"}"
  Subsystem53 : Subsystem
      settings: PortSchema="{\"entries\":[{\"content\":{\"sides\":[{\"content\":{\"connectorIds\":[\"In1\",\"In2\",\"In3\",\"In4\",\"In5\",\"In6\"]},\"type\":\"ConnectorPlacement.EquallySpacedRectSide\",\"uuid\":\"ec6071b1-e44d-45a4-9204-34cda7b2c9be\"},{\"content\":{\"side\":\"RIGHT\"},\"type\":\"ConnectorPlacement.EquallySpacedRectSide\",\"uuid\":\"8ac2ba72-278d-4942-985d-63a53d830fa7\"},{\"content\":{\"connectorIds\":[\"LConn1\"],\"side\":\"TOP\"},\"type\":\"ConnectorPlacement.EquallySpacedRectSide\",\"uuid\":\"91abef48-6106-4bba-9094-b5b4c6d4927b\"},{\"content\":{\"connectorIds\":[\"RConn1\"],\"side\":\"BOTTOM\"},\"type\":\"ConnectorPlacement.EquallySpacedRectSide\",\"uuid\":\"2339e630-2664-445f-8cd2-24ead5b760e5\"}]},\"type\":\"ConnectorPlacement.EquallySpacedConnector\",\"uuid\":\"6b30c10d-3aac-43c1-96cb-d205f04f2f88\"}],\"packageUris\":[\"http://schema.mathworks.com/mf0/Connector/R2020b\"],\"version\":\"1.0\"}"
  To Workspace2 : ToWorkspace  VariableName=diode_string1_power_out  SampleTime=-1
      settings: Save2DSignal=2-D array (concatenate along first dimension)
  V1 : spsVoltageMeasurementLib/Voltage Measurement  PhasorSimulation=off  OutputType=Complex  PSBequivalent=0
  Variable DC Source1 : Subsystem
  powergui2 : spspowerguiLib/powergui  Priority=1  SimulationMode=Discrete  SampleTime=2.5e-3  frequency=60  Iterations=500  frequencyindice=0  Pbase=100e6  ErrMax=1e-4  UnitsV=kV  UnitsW=MW  buscounter=0  FunctionMessages=off  echomessages=off  EnableUseOfTLC=off  CurrentSourceSwitches=on  DisableSnubberDevices=on  DisableRonSwitches=off  DisableVfSwitches=off  DisplayEquations=off  AutomaticDiscreteSolvers=off  SolverType=Tustin/Backward Euler (TBE)  Interpol=off  ExternalGateDelay=off  methode=off  Ts=0  x0status=blocks  SPID=off  SwTol=0  HookPort=off  NonlinearTolerance=1e-4  nMaxIteration=1000  ContinueOnMaxIteration=off  RestoreLinks=warning  ResistiveCurrentMeasurement=off  Frange=[0:2:500]  Ylog=off  Xlog=on  ShowGrid=off  save=off  variable=ZData  structure=0  ZoomFFT=on  StartTime=0.0  cycles=1  DisplayStyle=1  fundamental=60  FreqAxis=off  MaxFrequency=1000  frequencyindicesteady=1  RmsSteady=1  display=off
  Array Plot : ArrayPlot  IOType=viewer  WindowPosition=[117.000000,351.000000,800.000000,450.000000,]  ScopeFrameLocation=window  AxesScaling=Manual  YLimits=[-1,1]
  Scope{,1..3} (4 alike) : Scope
  wires:
  V1/1 -> Product2/2
  Product2/1 -> To Workspace2/1
  I1/1 -> Product2/1
  From Workspace2/1 -> Demux2/1
  Demux2/1 -> Subsystem12/1(Irr)
  Demux2/2 -> Subsystem12/2(Irr1)
  Demux2/3 -> Subsystem12/3(Irr2)
  Demux2/4 -> Subsystem12/4(Irr3)
  Demux2/5 -> Subsystem13/1(Irr)
  Demux2/6 -> Subsystem13/2(Irr1)
  Demux2/7 -> Subsystem13/3(Irr2)
  Demux2/8 -> Subsystem13/4(Irr3)
  Demux2/9 -> Subsystem13/5(Irr4)
  Demux2/10 -> Subsystem14/1(Irr)
  Demux2/11 -> Subsystem14/2(Irr1)
  Demux2/12 -> Subsystem14/3(Irr3)
  Demux2/13 -> Subsystem14/4(Irr4)
  Demux2/14 -> Subsystem14/5(Irr2)
  Demux2/15 -> Subsystem14/6(Irr5)
  Demux2/16 -> Subsystem15/1(Irr)
  Demux2/17 -> Subsystem15/2(Irr1)
  Demux2/18 -> Subsystem15/3(Irr2)
  Demux2/19 -> Subsystem15/4(Irr3)
  Demux2/20 -> Subsystem15/5(Irr4)
  Demux2/21 -> Subsystem15/6(Irr5)
  Demux2/22 -> Subsystem15/7(Irr6)
  Demux2/23 -> Subsystem16/1(Irr)
  Demux2/24 -> Subsystem16/2(Irr1)
  Demux2/25 -> Subsystem16/3(Irr2)
  Demux2/26 -> Subsystem16/4(Irr3)
  Demux2/27 -> Subsystem16/5(Irr4)
  Demux2/28 -> Subsystem16/6(Irr5)
  Demux2/29 -> Subsystem16/7(Irr6)
  Demux2/30 -> Subsystem17/1(Irr)
  Demux2/31 -> Subsystem17/2(Irr1)
  Demux2/32 -> Subsystem17/3(Irr2)
  Demux2/33 -> Subsystem17/4(Irr3)
  Demux2/34 -> Subsystem18/1(Irr)
  Demux2/35 -> Subsystem18/2(Irr1)
  Demux2/36 -> Subsystem18/3(Irr2)
  Demux2/37 -> Subsystem18/4(Irr3)
  Demux2/38 -> Subsystem19/1(Irr)
  Demux2/39 -> Subsystem19/2(Irr1)
  Demux2/40 -> Subsystem19/3(Irr2)
  Demux2/41 -> Subsystem19/4(Irr3)
  Demux2/42 -> Subsystem20/1(Irr)
  Demux2/43 -> Subsystem20/2(Irr1)
  Demux2/44 -> Subsystem20/3(Irr2)
  Demux2/45 -> Subsystem20/4(Irr3)
  Demux2/46 -> Subsystem34/1(Irr)
  Demux2/47 -> Subsystem34/2(Irr1)
  Demux2/48 -> Subsystem34/3(Irr2)
  Demux2/49 -> Subsystem34/4(Irr3)
  Demux2/50 -> Subsystem35/1(Irr)
  Demux2/51 -> Subsystem35/2(Irr1)
  Demux2/52 -> Subsystem35/3(Irr2)
  Demux2/53 -> Subsystem35/4(Irr3)
  Demux2/54 -> Subsystem36/1(Irr)
  Demux2/55 -> Subsystem36/2(Irr1)
  Demux2/56 -> Subsystem36/3(Irr2)
  Demux2/57 -> Subsystem36/4(Irr3)
  Demux2/58 -> Subsystem37/1(Irr)
  Demux2/59 -> Subsystem37/2(Irr1)
  Demux2/60 -> Subsystem37/3(Irr2)
  Demux2/61 -> Subsystem37/4(Irr3)
  Demux2/62 -> Subsystem37/5(Irr4)
  Demux2/63 -> Subsystem38/1(Irr)
  Demux2/64 -> Subsystem38/2(Irr1)
  Demux2/65 -> Subsystem38/3(Irr2)
  Demux2/66 -> Subsystem38/4(Irr3)
  Demux2/67 -> Subsystem39/1(Irr)
  Demux2/68 -> Subsystem39/2(Irr1)
  Demux2/69 -> Subsystem39/3(Irr2)
  Demux2/70 -> Subsystem39/4(Irr3)
  Demux2/71 -> Subsystem39/5(Irr4)
  Demux2/72 -> Subsystem40/1(Irr)
  Demux2/73 -> Subsystem40/2(Irr1)
  Demux2/74 -> Subsystem40/3(Irr2)
  Demux2/75 -> Subsystem40/4(Irr3)
  Demux2/76 -> Subsystem41/1(Irr)
  Demux2/77 -> Subsystem41/2(Irr1)
  Demux2/78 -> Subsystem41/3(Irr2)
  Demux2/79 -> Subsystem41/4(Irr3)
  Demux2/80 -> Subsystem41/5(Irr4)
  Demux2/81 -> Subsystem42/1(Irr)
  Demux2/82 -> Subsystem42/2(Irr1)
  Demux2/83 -> Subsystem42/3(Irr2)
  Demux2/84 -> Subsystem42/4(Irr3)
  Demux2/85 -> Subsystem43/1(Irr)
  Demux2/86 -> Subsystem43/2(Irr1)
  Demux2/87 -> Subsystem43/3(Irr2)
  Demux2/88 -> Subsystem43/4(Irr3)
  Demux2/89 -> Subsystem43/5(Irr4)
  Demux2/90 -> Subsystem44/1(Irr)
  Demux2/91 -> Subsystem44/2(Irr1)
  Demux2/92 -> Subsystem44/3(Irr2)
  Demux2/93 -> Subsystem44/4(Irr3)
  Demux2/94 -> Subsystem45/1(Irr)
  Demux2/95 -> Subsystem45/2(Irr1)
  Demux2/96 -> Subsystem45/3(Irr2)
  Demux2/97 -> Subsystem45/4(Irr3)
  Demux2/98 -> Subsystem45/5(Irr4)
  Demux2/99 -> Subsystem46/1(Irr)
  Demux2/100 -> Subsystem46/2(Irr1)
  Demux2/101 -> Subsystem46/3(Irr2)
  Demux2/102 -> Subsystem46/4(Irr3)
  Demux2/103 -> Subsystem46/5(Irr4)
  Demux2/104 -> Subsystem47/1(Irr)
  Demux2/105 -> Subsystem47/2(Irr1)
  Demux2/106 -> Subsystem47/3(Irr3)
  Demux2/107 -> Subsystem47/4(Irr4)
  Demux2/108 -> Subsystem47/5(Irr2)
  Demux2/109 -> Subsystem47/6(Irr5)
  Demux2/110 -> Subsystem48/1(Irr)
  Demux2/111 -> Subsystem48/2(Irr1)
  Demux2/112 -> Subsystem48/3(Irr2)
  Demux2/113 -> Subsystem48/4(Irr3)
  Demux2/114 -> Subsystem48/5(Irr4)
  Demux2/115 -> Subsystem49/1(Irr)
  Demux2/116 -> Subsystem49/2(Irr1)
  Demux2/117 -> Subsystem49/3(Irr3)
  Demux2/118 -> Subsystem49/4(Irr4)
  Demux2/119 -> Subsystem49/5(Irr2)
  Demux2/120 -> Subsystem49/6(Irr5)
  Demux2/121 -> Subsystem50/1(Irr)
  Demux2/122 -> Subsystem50/2(Irr1)
  Demux2/123 -> Subsystem50/3(Irr2)
  Demux2/124 -> Subsystem50/4(Irr3)
  Demux2/125 -> Subsystem50/5(Irr4)
  Demux2/126 -> Subsystem51/1(Irr)
  Demux2/127 -> Subsystem51/2(Irr1)
  Demux2/128 -> Subsystem51/3(Irr3)
  Demux2/129 -> Subsystem51/4(Irr4)
  Demux2/130 -> Subsystem51/5(Irr2)
  Demux2/131 -> Subsystem51/6(Irr5)
  Demux2/132 -> Subsystem52/1(Irr)
  Demux2/133 -> Subsystem52/2(Irr1)
  Demux2/134 -> Subsystem52/3(Irr2)
  Demux2/135 -> Subsystem52/4(Irr3)
  Demux2/136 -> Subsystem52/5(Irr4)
  Demux2/137 -> Subsystem53/1(Irr)
  Demux2/138 -> Subsystem53/2(Irr1)
  Demux2/139 -> Subsystem53/3(Irr3)
  Demux2/140 -> Subsystem53/4(Irr4)
  Demux2/141 -> Subsystem53/5(Irr2)
  Demux2/142 -> Subsystem53/6(Irr5)
  connections:
  Variable DC Source1/LConn1 -- I1/RConn1 -- V1/LConn1
  Subsystem53/RConn1 -- Variable DC Source1/LConn2 -- V1/LConn2 -- Bypass Diode 53/LConn1
  Subsystem12/LConn1 -- I1/LConn1 -- Bypass Diode 12/RConn1
  Subsystem13/LConn1 -- Bypass Diode 12/LConn1 -- Subsystem12/RConn1 -- Bypass Diode 13/RConn1
  Subsystem14/LConn1 -- Bypass Diode 13/LConn1 -- Subsystem13/RConn1 -- Bypass Diode 14/RConn1
  Subsystem15/LConn1 -- Bypass Diode 14/LConn1 -- Subsystem14/RConn1 -- Bypass Diode 15/RConn1
  Subsystem16/LConn1 -- Bypass Diode 15/LConn1 -- Subsystem15/RConn1 -- Bypass Diode 16/RConn1
  Subsystem17/LConn1 -- Subsystem16/RConn1 -- Bypass Diode 16/LConn1 -- Bypass Diode 17/RConn1
  Subsystem18/LConn1 -- Subsystem17/RConn1 -- Bypass Diode 17/LConn1 -- Bypass Diode 18/RConn1
  Subsystem19/LConn1 -- Subsystem18/RConn1 -- Bypass Diode 18/LConn1 -- Bypass Diode 19/RConn1
  Bypass Diode 19/LConn1 -- Bypass Diode 20/RConn1 -- Subsystem20/LConn1 -- Subsystem19/RConn1
  Subsystem34/LConn1 -- Subsystem20/RConn1 -- Bypass Diode 20/LConn1 -- Bypass Diode 34/RConn1
  Bypass Diode 34/LConn1 -- Bypass Diode 35/RConn1 -- Subsystem35/LConn1 -- Subsystem34/RConn1
  Subsystem37/LConn1 -- Subsystem36/RConn1 -- Bypass Diode 36/LConn1 -- Bypass Diode 37/RConn1
  Bypass Diode 35/LConn1 -- Bypass Diode 36/RConn1 -- Subsystem36/LConn1 -- Subsystem35/RConn1
  Subsystem38/LConn1 -- Bypass Diode 37/LConn1 -- Subsystem37/RConn1 -- Bypass Diode 38/RConn1
  Subsystem39/LConn1 -- Subsystem38/RConn1 -- Bypass Diode 38/LConn1 -- Bypass Diode 39/RConn1
  Subsystem40/LConn1 -- Bypass Diode 40/RConn1 -- Bypass Diode 39/LConn1 -- Subsystem39/RConn1
  Subsystem41/LConn1 -- Bypass Diode 41/RConn1 -- Subsystem40/RConn1 -- Bypass Diode 40/LConn1
  Subsystem42/LConn1 -- Bypass Diode 42/RConn1 -- Bypass Diode 41/LConn1 -- Subsystem41/RConn1
  Bypass Diode 42/LConn1 -- Subsystem42/RConn1 -- Bypass Diode 43/RConn1 -- Subsystem43/LConn1
  Subsystem44/LConn1 -- Bypass Diode 44/RConn1 -- Bypass Diode 43/LConn1 -- Subsystem43/RConn1
  Bypass Diode 44/LConn1 -- Subsystem44/RConn1 -- Bypass Diode 45/RConn1 -- Subsystem45/LConn1
  Subsystem46/LConn1 -- Bypass Diode 45/LConn1 -- Subsystem45/RConn1 -- Bypass Diode 46/RConn1
  Subsystem47/LConn1 -- Bypass Diode 46/LConn1 -- Subsystem46/RConn1 -- Bypass Diode 47/RConn1
  Subsystem48/LConn1 -- Subsystem47/RConn1 -- Bypass Diode 47/LConn1 -- Bypass Diode 48/RConn1
  Subsystem48/RConn1 -- Subsystem49/LConn1 -- Bypass Diode 49/RConn1 -- Bypass Diode 48/LConn1
  Subsystem50/LConn1 -- Bypass Diode 49/LConn1 -- Subsystem49/RConn1 -- Bypass Diode 50/RConn1
  Bypass Diode 50/LConn1 -- Subsystem50/RConn1 -- Subsystem51/LConn1 -- Bypass Diode 51/RConn1
  Subsystem52/LConn1 -- Bypass Diode 51/LConn1 -- Subsystem51/RConn1 -- Bypass Diode 52/RConn1
  Bypass Diode 52/LConn1 -- Subsystem52/RConn1 -- Subsystem53/LConn1 -- Bypass Diode 53/RConn1

== system DV3A_String1_Diode/Subsystem12 ==
  Irr : Inport
  Irr1 : Inport  Port=2
  Irr2 : Inport  Port=3
  Irr3 : Inport  Port=4
  PV1 : Subsystem
      settings: PortSchema="{\"entries\":[{\"content\":{\"sides\":[{\"content\":{\"connectorIds\":[\"In1\"]},\"type\":\"ConnectorPlacement.EquallySpacedRectSide\",\"uuid\":\"5c508248-bd07-48d5-951d-be180bcc8740\"},{\"content\":{\"connectorIds\":[],\"side\":\"RIGHT\"},\"type\":\"ConnectorPlacement.EquallySpacedRectSide\",\"uuid\":\"e31a9bdc-b533-497f-8610-a92a4eef02bc\"},{\"content\":{\"connectorIds\":[\"LConn1\"],\"side\":\"TOP\"},\"type\":\"ConnectorPlacement.EquallySpacedRectSide\",\"uuid\":\"a80efd6c-0c74-41ec-a161-3d709011a457\"},{\"content\":{\"connectorIds\":[\"RConn1\"],\"side\":\"BOTTOM\"},\"type\":\"ConnectorPlacement.EquallySpacedRectSide\",\"uuid\":\"e2d028a7-872a-45fc-84e4-cb840db01281\"}]},\"type\":\"ConnectorPlacement.EquallySpacedConnector\",\"uuid\":\"57d442c0-d58c-4dd4-aeba-72d113e063d7\"}],\"packageUris\":[\"http://schema.mathworks.com/mf0/Connector/19700101\"],\"version\":\"1.0\"}"
  PV2 : Subsystem
      settings: PortSchema="{\"entries\":[{\"content\":{\"sides\":[{\"content\":{\"connectorIds\":[\"In1\"]},\"type\":\"ConnectorPlacement.EquallySpacedRectSide\",\"uuid\":\"5c508248-bd07-48d5-951d-be180bcc8740\"},{\"content\":{\"connectorIds\":[],\"side\":\"RIGHT\"},\"type\":\"ConnectorPlacement.EquallySpacedRectSide\",\"uuid\":\"e31a9bdc-b533-497f-8610-a92a4eef02bc\"},{\"content\":{\"connectorIds\":[\"LConn1\"],\"side\":\"TOP\"},\"type\":\"ConnectorPlacement.EquallySpacedRectSide\",\"uuid\":\"a80efd6c-0c74-41ec-a161-3d709011a457\"},{\"content\":{\"connectorIds\":[\"RConn1\"],\"side\":\"BOTTOM\"},\"type\":\"ConnectorPlacement.EquallySpacedRectSide\",\"uuid\":\"e2d028a7-872a-45fc-84e4-cb840db01281\"}]},\"type\":\"ConnectorPlacement.EquallySpacedConnector\",\"uuid\":\"57d442c0-d58c-4dd4-aeba-72d113e063d7\"}],\"packageUris\":[\"http://schema.mathworks.com/mf0/Connector/19700101\"],\"version\":\"1.0\"}"
  PV3 : Subsystem
      settings: PortSchema="{\"entries\":[{\"content\":{\"sides\":[{\"content\":{\"connectorIds\":[\"In1\"]},\"type\":\"ConnectorPlacement.EquallySpacedRectSide\",\"uuid\":\"5c508248-bd07-48d5-951d-be180bcc8740\"},{\"content\":{\"connectorIds\":[],\"side\":\"RIGHT\"},\"type\":\"ConnectorPlacement.EquallySpacedRectSide\",\"uuid\":\"e31a9bdc-b533-497f-8610-a92a4eef02bc\"},{\"content\":{\"connectorIds\":[\"LConn1\"],\"side\":\"TOP\"},\"type\":\"ConnectorPlacement.EquallySpacedRectSide\",\"uuid\":\"a80efd6c-0c74-41ec-a161-3d709011a457\"},{\"content\":{\"connectorIds\":[\"RConn1\"],\"side\":\"BOTTOM\"},\"type\":\"ConnectorPlacement.EquallySpacedRectSide\",\"uuid\":\"e2d028a7-872a-45fc-84e4-cb840db01281\"}]},\"type\":\"ConnectorPlacement.EquallySpacedConnector\",\"uuid\":\"57d442c0-d58c-4dd4-aeba-72d113e063d7\"}],\"packageUris\":[\"http://schema.mathworks.com/mf0/Connector/19700101\"],\"version\":\"1.0\"}"
  PV4 : Subsystem
      settings: PortSchema="{\"entries\":[{\"content\":{\"sides\":[{\"content\":{\"connectorIds\":[\"In1\"]},\"type\":\"ConnectorPlacement.EquallySpacedRectSide\",\"uuid\":\"5c508248-bd07-48d5-951d-be180bcc8740\"},{\"content\":{\"connectorIds\":[],\"side\":\"RIGHT\"},\"type\":\"ConnectorPlacement.EquallySpacedRectSide\",\"uuid\":\"e31a9bdc-b533-497f-8610-a92a4eef02bc\"},{\"content\":{\"connectorIds\":[\"LConn1\"],\"side\":\"TOP\"},\"type\":\"ConnectorPlacement.EquallySpacedRectSide\",\"uuid\":\"a80efd6c-0c74-41ec-a161-3d709011a457\"},{\"content\":{\"connectorIds\":[\"RConn1\"],\"side\":\"BOTTOM\"},\"type\":\"ConnectorPlacement.EquallySpacedRectSide\",\"uuid\":\"e2d028a7-872a-45fc-84e4-cb840db01281\"}]},\"type\":\"ConnectorPlacement.EquallySpacedConnector\",\"uuid\":\"57d442c0-d58c-4dd4-aeba-72d113e063d7\"}],\"packageUris\":[\"http://schema.mathworks.com/mf0/Connector/19700101\"],\"version\":\"1.0\"}"
  + : PMIOPort  Side=Left
  - : PMIOPort  Port=2  Side=Right
  wires:
  Irr2/1 -> PV1/1(Irr)
  Irr/1 -> PV2/1(Irr)
  Irr1/1 -> PV4/1(Irr)
  Irr3/1 -> PV3/1(Irr)
  connections:
  PV2/LConn1 -- +/RConn1
  PV4/RConn1 -- PV1/LConn1
  PV4/LConn1 -- PV2/RConn1
  PV3/RConn1 -- -/RConn1
  PV1/RConn1 -- PV3/LConn1
